simulink model "v19_POA"  (R2023a)
settings: Solver=ode1  StartTime=0.0  StopTime=86400  FixedStep=4  RelTol=1e-3
settings Model: Creator=poupelel  LastModifiedBy=Solal
settings SolverCC: AlgebraicLoopSolver=TrustRegion
settings DebuggingCC: UnconnectedInputMsg=warning  UnconnectedOutputMsg=warning  UnconnectedLineMsg=warning
settings ModelReferenceCC: EnableRefExpFcnMdlSchedulingChecks=on
settings RTWCC: DLArmComputeVersion=19.05

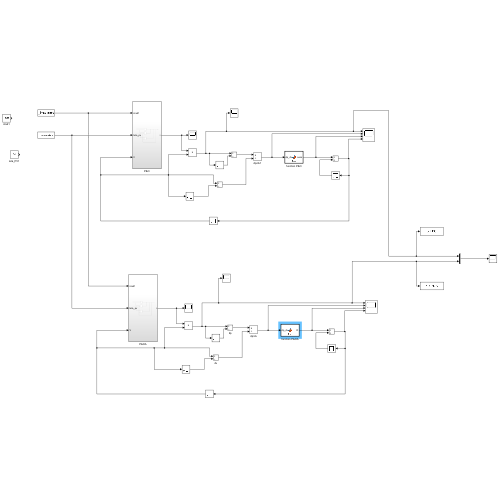
[thumbnail: Simulink's stored preview of the top-level diagram]
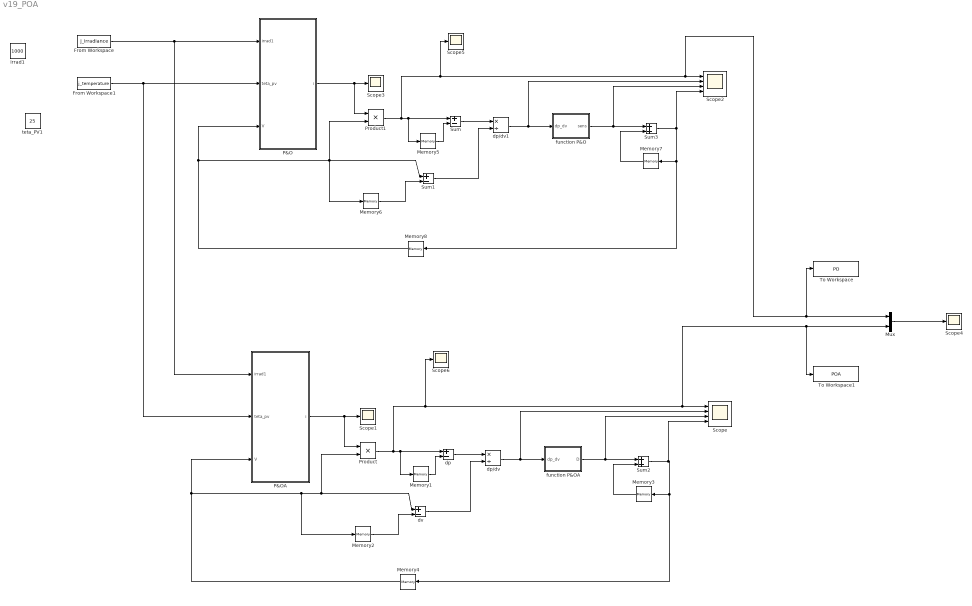
== system v19_POA ==
  From Workspace : FromWorkspace  VariableName=j_irradiance
  From Workspace1 : FromWorkspace  VariableName=j_temperature
  Memory{1..8} (8 alike) : Memory
  Mux : Mux  Inputs=2
  P&O : Subsystem
  P&OA : Subsystem
  Product : Product
  Product1 : Product
  Scope : Scope  NumInputPorts=4
  Scope{1,3..6} (5 alike) : Scope
  Scope2 : Scope  NumInputPorts=4
  Sum : Sum  Inputs=+-
  Sum1 : Sum  Inputs=+-
  Sum2 : Sum
  Sum3 : Sum
  To Workspace : ToWorkspace  VariableName=PO  SampleTime=-1
  To Workspace1 : ToWorkspace  VariableName=POA  SampleTime=-1
  dp : Sum  Inputs=+-
  dp/dv : Product  Inputs=*/
  dp/dv1 : Product  Inputs=*/
  dv : Sum  Inputs=+-
  function P&O : MATLAB Function  TreatAsAtomicUnit=on
  function P&OA : MATLAB Function  TreatAsAtomicUnit=on
  irrad1 : Constant  Value=1000
  teta_PV1 : Constant  Value=25
  wires:
  From Workspace/1 -> P&OA/1(irrad1), P&O/1(irrad1)
  From Workspace1/1 -> P&OA/2(teta_pv), P&O/2(teta_pv)
  Memory1/1 -> dp/2
  dp/1 -> dp/dv/1
  Memory2/1 -> dv/2
  dv/1 -> dp/dv/2
  dp/dv/1 -> Scope/2, function P&OA/1(dp_dv)
  Product/1 -> Scope6/1, To Workspace1/1, Mux/2, Scope/1, Memory1/1, dp/1
  function P&OA/1(D) -> Scope/3, Sum2/1
  Sum2/1 -> Scope/4, Memory3/1, Memory4/1
  Memory3/1 -> Sum2/2
  Sum3/1 -> Scope2/4, Memory7/1, Memory8/1
  Memory7/1 -> Sum3/2
  function P&O/1(sens) -> Scope2/3, Sum3/1
  Sum/1 -> dp/dv1/1
  Product1/1 -> Scope5/1, Scope2/1, To Workspace/1, Mux/1, Memory5/1, Sum/1
  Memory5/1 -> Sum/2
  Sum1/1 -> dp/dv1/2
  dp/dv1/1 -> Scope2/2, function P&O/1(dp_dv)
  Memory6/1 -> Sum1/2
  Mux/1 -> Scope4/1
  P&O/1(i) -> Scope3/1, Product1/1
  P&OA/1(i) -> Product/1, Scope1/1
  Memory4/1 -> P&OA/3(V), dv/1, Product/2, Memory2/1
  Memory8/1 -> P&O/3(V), Sum1/1, Product1/2, Memory6/1

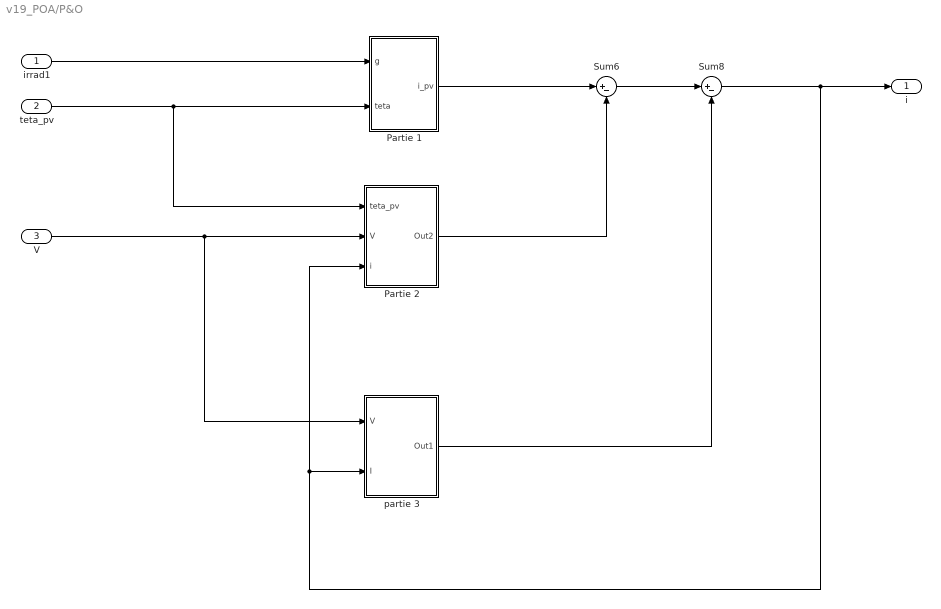
== system v19_POA/P&O ==
  irrad1 : Inport
  teta_pv : Inport  Port=2
  V : Inport  Port=3
  Partie 1 : Subsystem
  Partie 2 : Subsystem
  Sum6 : Sum  Inputs=|+-
  Sum8 : Sum  Inputs=|+-
  partie 3 : Subsystem
  i : Outport
  wires:
  Partie 1/1(i_pv) -> Sum6/1
  teta_pv/1 -> Partie 2/1(teta_pv), Partie 1/2(teta)
  Sum6/1 -> Sum8/1
  Sum8/1 -> i/1, Partie 2/3(i), partie 3/2(I)
  irrad1/1 -> Partie 1/1(g)
  V/1 -> partie 3/1(V), Partie 2/2(V)
  Partie 2/1(Out2) -> Sum6/2
  partie 3/1(Out1) -> Sum8/2

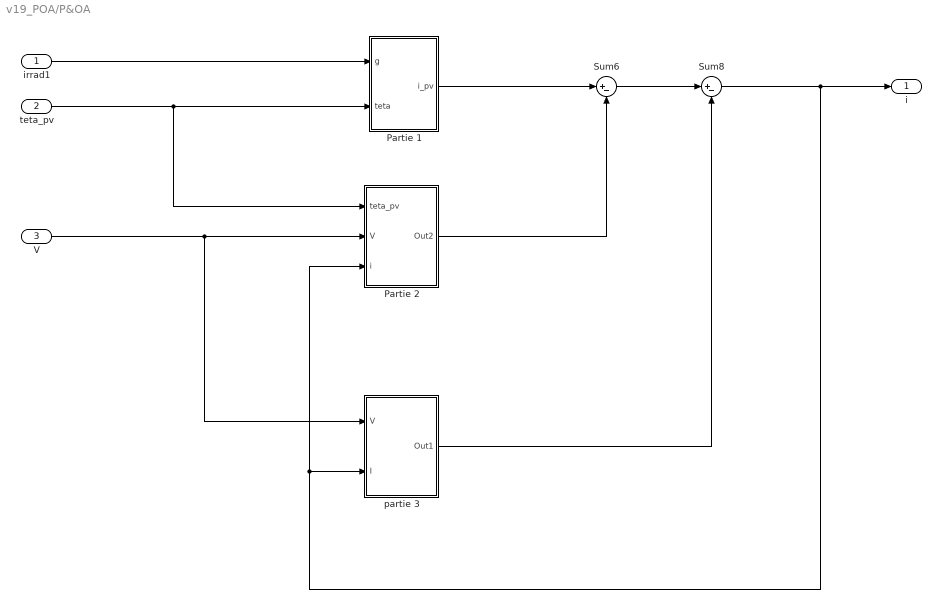
== system v19_POA/P&OA ==
  irrad1 : Inport
  teta_pv : Inport  Port=2
  V : Inport  Port=3
  Partie 1 : Subsystem
  Partie 2 : Subsystem
  Sum6 : Sum  Inputs=|+-
  Sum8 : Sum  Inputs=|+-
  partie 3 : Subsystem
  i : Outport
  wires:
  Partie 1/1(i_pv) -> Sum6/1
  teta_pv/1 -> Partie 2/1(teta_pv), Partie 1/2(teta)
  Sum6/1 -> Sum8/1
  Sum8/1 -> i/1, Partie 2/3(i), partie 3/2(I)
  irrad1/1 -> Partie 1/1(g)
  V/1 -> partie 3/1(V), Partie 2/2(V)
  Partie 2/1(Out2) -> Sum6/2
  partie 3/1(Out1) -> Sum8/2

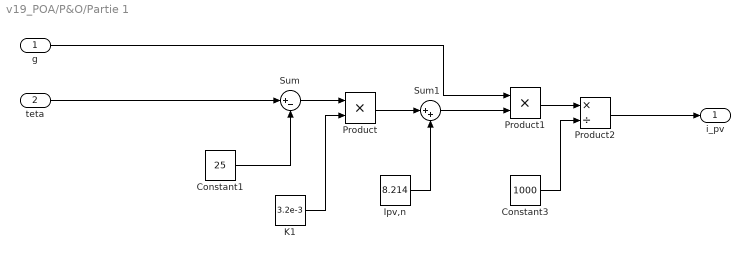
== system v19_POA/P&O/Partie 1 ==
  g : Inport
  teta : Inport  Port=2
  Constant1 : Constant  Value=25
  Constant3 : Constant  Value=1000
  Ipv,n : Constant  Value=8.214
  K1 : Constant  Value=3.2e-3
  Product : Product
  Product1 : Product
  Product2 : Product  Inputs=*/
  Sum : Sum  Inputs=|+-
  Sum1 : Sum  Inputs=|++
  i_pv : Outport
  wires:
  Ipv,n/1 -> Sum1/2
  Sum1/1 -> Product1/2
  Constant3/1 -> Product2/2
  K1/1 -> Product/2
  Constant1/1 -> Sum/2
  Sum/1 -> Product/1
  Product1/1 -> Product2/1
  Product2/1 -> i_pv/1
  Product/1 -> Sum1/1
  teta/1 -> Sum/1
  g/1 -> Product1/1

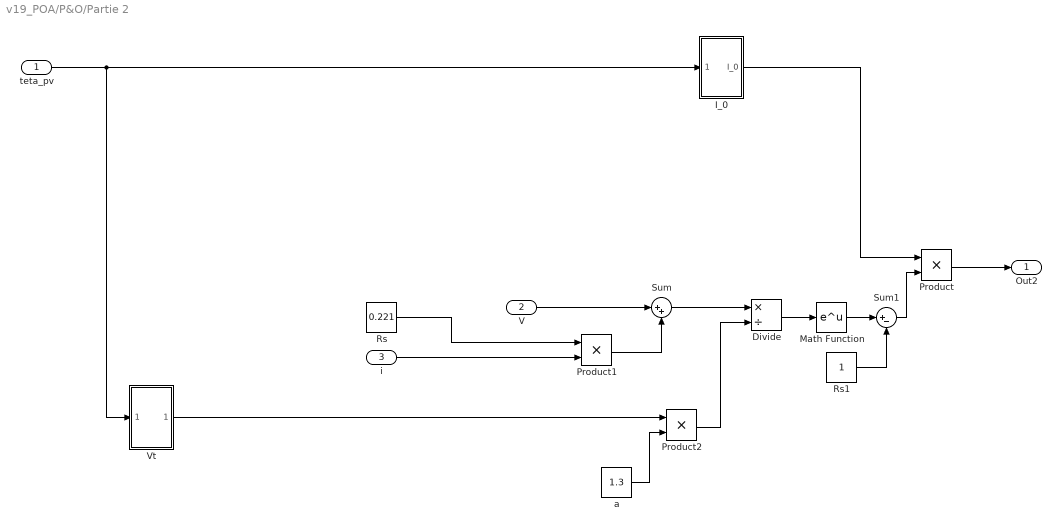
== system v19_POA/P&O/Partie 2 ==
  teta_pv : Inport
  V : Inport  Port=2
  i : Inport  Port=3
  Divide : Product  Inputs=*/
  I_0 : Subsystem
  Math Function : Math
  Product : Product
  Product1 : Product
  Product2 : Product
  Rs : Constant  Value=0.221
  Rs1 : Constant
  Sum : Sum  Inputs=|++
  Sum1 : Sum  Inputs=|+-
  Vt : Subsystem
  a : Constant  Value=1.3
  Out2 : Outport
  wires:
  Sum1/1 -> Product/2
  Rs/1 -> Product1/1
  Vt/1(Out1) -> Product2/1
  Math Function/1 -> Sum1/1
  Divide/1 -> Math Function/1
  V/1 -> Sum/1
  Product2/1 -> Divide/2
  I_0/1(I_0) -> Product/1
  Sum/1 -> Divide/1
  teta_pv/1 -> I_0/1(teta), Vt/1(teta_pv)
  a/1 -> Product2/2
  Product1/1 -> Sum/2
  i/1 -> Product1/2
  Rs1/1 -> Sum1/2
  Product/1 -> Out2/1

== system v19_POA/P&O/partie 3 ==
  V : Inport
  I : Inport  Port=2
  Divide : Product  Inputs=*/
  Product : Product
  Rp : Constant  Value=415.4
  Rs : Constant  Value=0.221
  Sum : Sum  Inputs=|++
  Out1 : Outport
  wires:
  Sum/1 -> Divide/1
  I/1 -> Product/1
  Rp/1 -> Divide/2
  Product/1 -> Sum/1
  Divide/1 -> Out1/1
  Rs/1 -> Product/2
  V/1 -> Sum/2

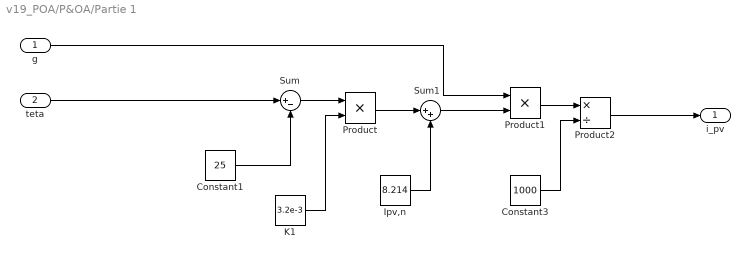
== system v19_POA/P&OA/Partie 1 ==
  g : Inport
  teta : Inport  Port=2
  Constant1 : Constant  Value=25
  Constant3 : Constant  Value=1000
  Ipv,n : Constant  Value=8.214
  K1 : Constant  Value=3.2e-3
  Product : Product
  Product1 : Product
  Product2 : Product  Inputs=*/
  Sum : Sum  Inputs=|+-
  Sum1 : Sum  Inputs=|++
  i_pv : Outport
  wires:
  Ipv,n/1 -> Sum1/2
  Sum1/1 -> Product1/2
  Constant3/1 -> Product2/2
  K1/1 -> Product/2
  Constant1/1 -> Sum/2
  Sum/1 -> Product/1
  Product1/1 -> Product2/1
  Product2/1 -> i_pv/1
  Product/1 -> Sum1/1
  teta/1 -> Sum/1
  g/1 -> Product1/1

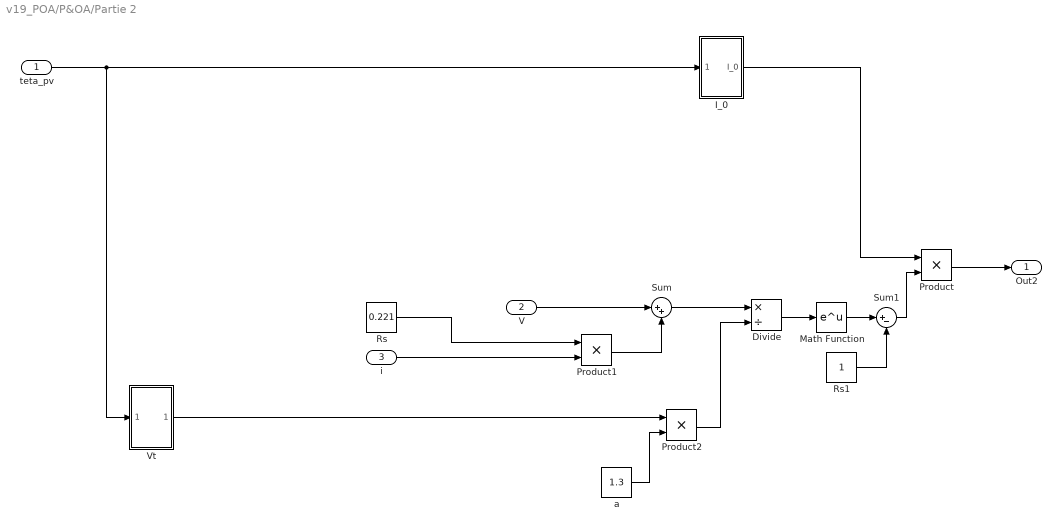
== system v19_POA/P&OA/Partie 2 ==
  teta_pv : Inport
  V : Inport  Port=2
  i : Inport  Port=3
  Divide : Product  Inputs=*/
  I_0 : Subsystem
  Math Function : Math
  Product : Product
  Product1 : Product
  Product2 : Product
  Rs : Constant  Value=0.221
  Rs1 : Constant
  Sum : Sum  Inputs=|++
  Sum1 : Sum  Inputs=|+-
  Vt : Subsystem
  a : Constant  Value=1.3
  Out2 : Outport
  wires:
  Sum1/1 -> Product/2
  Rs/1 -> Product1/1
  Vt/1(Out1) -> Product2/1
  Math Function/1 -> Sum1/1
  Divide/1 -> Math Function/1
  V/1 -> Sum/1
  Product2/1 -> Divide/2
  I_0/1(I_0) -> Product/1
  Sum/1 -> Divide/1
  teta_pv/1 -> I_0/1(teta), Vt/1(teta_pv)
  a/1 -> Product2/2
  Product1/1 -> Sum/2
  i/1 -> Product1/2
  Rs1/1 -> Sum1/2
  Product/1 -> Out2/1

== system v19_POA/P&OA/partie 3 ==
  V : Inport
  I : Inport  Port=2
  Divide : Product  Inputs=*/
  Product : Product
  Rp : Constant  Value=415.4
  Rs : Constant  Value=0.221
  Sum : Sum  Inputs=|++
  Out1 : Outport
  wires:
  Sum/1 -> Divide/1
  I/1 -> Product/1
  Rp/1 -> Divide/2
  Product/1 -> Sum/1
  Divide/1 -> Out1/1
  Rs/1 -> Product/2
  V/1 -> Sum/2

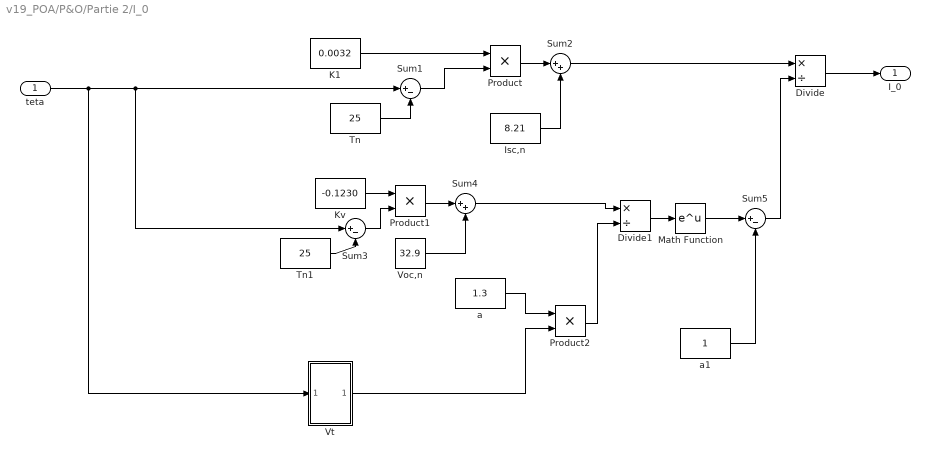
== system v19_POA/P&O/Partie 2/I_0 ==
  teta : Inport
  Divide : Product  Inputs=*/
  Divide1 : Product  Inputs=*/
  Isc,n : Constant  Value=8.21
  K1 : Constant  Value=0.0032
  Kv : Constant  Value=-0.1230
  Math Function : Math
  Product : Product
  Product1 : Product
  Product2 : Product
  Sum1 : Sum  Inputs=|+-
  Sum2 : Sum  Inputs=|++
  Sum3 : Sum  Inputs=|+-
  Sum4 : Sum  Inputs=|++
  Sum5 : Sum  Inputs=|+-
  Tn : Constant  Value=25
  Tn1 : Constant  Value=25
  Voc,n : Constant  Value=32.9
  Vt : Subsystem
  a : Constant  Value=1.3
  a1 : Constant
  I_0 : Outport
  wires:
  Sum3/1 -> Product1/2
  a/1 -> Product2/1
  Kv/1 -> Product1/1
  teta/1 -> Vt/1(In1), Sum3/1, Sum1/1
  Voc,n/1 -> Sum4/2
  Sum2/1 -> Divide/1
  Product1/1 -> Sum4/1
  K1/1 -> Product/1
  Sum1/1 -> Product/2
  Vt/1(Out1) -> Product2/2
  Tn/1 -> Sum1/2
  Isc,n/1 -> Sum2/2
  Product/1 -> Sum2/1
  Product2/1 -> Divide1/2
  Tn1/1 -> Sum3/2
  Sum5/1 -> Divide/2
  a1/1 -> Sum5/2
  Divide/1 -> I_0/1
  Sum4/1 -> Divide1/1
  Divide1/1 -> Math Function/1
  Math Function/1 -> Sum5/1

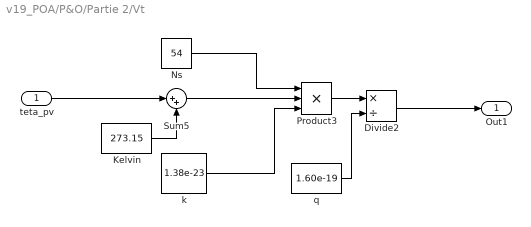
== system v19_POA/P&O/Partie 2/Vt ==
  teta_pv : Inport
  Divide2 : Product  Inputs=*/
  Kelvin : Constant  Value=273.15
  Ns : Constant  Value=54
  Product3 : Product  Inputs=3
  Sum5 : Sum  Inputs=|++
  k : Constant  Value=1.38e-23
  q : Constant  Value=1.60e-19
  Out1 : Outport
  wires:
  q/1 -> Divide2/2
  Sum5/1 -> Product3/2
  k/1 -> Product3/3
  Product3/1 -> Divide2/1
  Ns/1 -> Product3/1
  Divide2/1 -> Out1/1
  teta_pv/1 -> Sum5/1
  Kelvin/1 -> Sum5/2

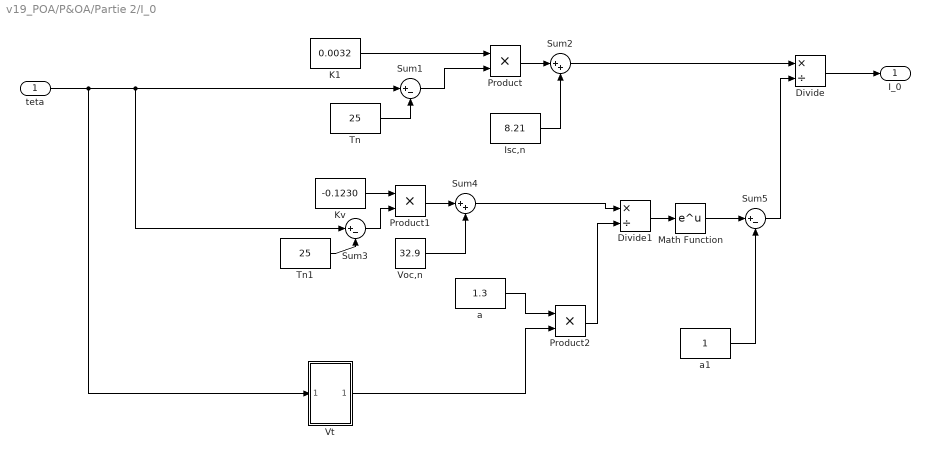
== system v19_POA/P&OA/Partie 2/I_0 ==
  teta : Inport
  Divide : Product  Inputs=*/
  Divide1 : Product  Inputs=*/
  Isc,n : Constant  Value=8.21
  K1 : Constant  Value=0.0032
  Kv : Constant  Value=-0.1230
  Math Function : Math
  Product : Product
  Product1 : Product
  Product2 : Product
  Sum1 : Sum  Inputs=|+-
  Sum2 : Sum  Inputs=|++
  Sum3 : Sum  Inputs=|+-
  Sum4 : Sum  Inputs=|++
  Sum5 : Sum  Inputs=|+-
  Tn : Constant  Value=25
  Tn1 : Constant  Value=25
  Voc,n : Constant  Value=32.9
  Vt : Subsystem
  a : Constant  Value=1.3
  a1 : Constant
  I_0 : Outport
  wires:
  Sum3/1 -> Product1/2
  a/1 -> Product2/1
  Kv/1 -> Product1/1
  teta/1 -> Vt/1(In1), Sum3/1, Sum1/1
  Voc,n/1 -> Sum4/2
  Sum2/1 -> Divide/1
  Product1/1 -> Sum4/1
  K1/1 -> Product/1
  Sum1/1 -> Product/2
  Vt/1(Out1) -> Product2/2
  Tn/1 -> Sum1/2
  Isc,n/1 -> Sum2/2
  Product/1 -> Sum2/1
  Product2/1 -> Divide1/2
  Tn1/1 -> Sum3/2
  Sum5/1 -> Divide/2
  a1/1 -> Sum5/2
  Divide/1 -> I_0/1
  Sum4/1 -> Divide1/1
  Divide1/1 -> Math Function/1
  Math Function/1 -> Sum5/1

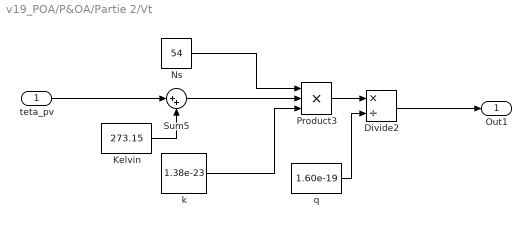
== system v19_POA/P&OA/Partie 2/Vt ==
  teta_pv : Inport
  Divide2 : Product  Inputs=*/
  Kelvin : Constant  Value=273.15
  Ns : Constant  Value=54
  Product3 : Product  Inputs=3
  Sum5 : Sum  Inputs=|++
  k : Constant  Value=1.38e-23
  q : Constant  Value=1.60e-19
  Out1 : Outport
  wires:
  q/1 -> Divide2/2
  Sum5/1 -> Product3/2
  k/1 -> Product3/3
  Product3/1 -> Divide2/1
  Ns/1 -> Product3/1
  Divide2/1 -> Out1/1
  teta_pv/1 -> Sum5/1
  Kelvin/1 -> Sum5/2

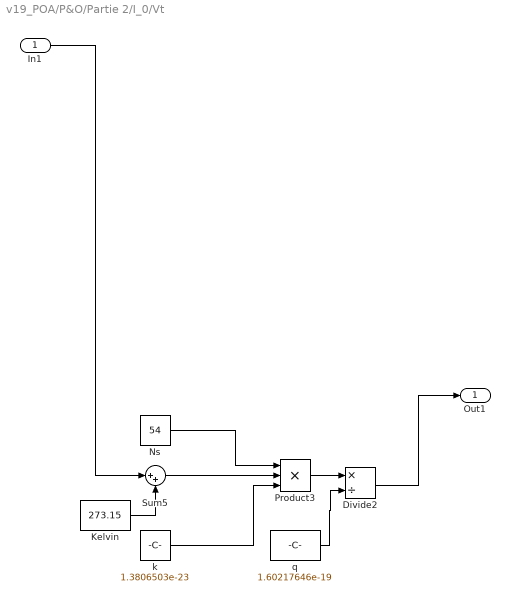
== system v19_POA/P&O/Partie 2/I_0/Vt ==
  In1 : Inport
  Divide2 : Product  Inputs=*/
  Kelvin : Constant  Value=273.15
  Ns : Constant  Value=54
  Product3 : Product  Inputs=3
  Sum5 : Sum  Inputs=|++
  k : Constant  Value=1.3806503e-23
  q : Constant  Value=1.60217646e-19
  Out1 : Outport
  wires:
  q/1 -> Divide2/2
  Sum5/1 -> Product3/2
  k/1 -> Product3/3
  Product3/1 -> Divide2/1
  Ns/1 -> Product3/1
  Divide2/1 -> Out1/1
  In1/1 -> Sum5/1
  Kelvin/1 -> Sum5/2

== system v19_POA/P&OA/Partie 2/I_0/Vt ==
  In1 : Inport
  Divide2 : Product  Inputs=*/
  Kelvin : Constant  Value=273.15
  Ns : Constant  Value=54
  Product3 : Product  Inputs=3
  Sum5 : Sum  Inputs=|++
  k : Constant  Value=1.3806503e-23
  q : Constant  Value=1.60217646e-19
  Out1 : Outport
  wires:
  q/1 -> Divide2/2
  Sum5/1 -> Product3/2
  k/1 -> Product3/3
  Product3/1 -> Divide2/1
  Ns/1 -> Product3/1
  Divide2/1 -> Out1/1
  In1/1 -> Sum5/1
  Kelvin/1 -> Sum5/2

== matlab function v19_POA/function P&OA ==
  data: dp_dv input; D output
function D=fcn(dp_dv)
dDbig=1
dDsmall=0.2
D=0
error=6
if dp_dv<error
    dD=dDbig
else
    dD=dDsmall
end
if dp_dv>0
        D=D+dD
    else
        D=D-dD
end

== matlab function v19_POA/function P&O ==
  data: dp_dv input; sens output
function sens = fcn(dp_dv)
if dp_dv<0
    sens=-1;
else 
    sens=1;
end
